simulink model "ReceiveAndUnpack"  (R2023b)
settings: Solver=FixedStepAuto  StartTime=0.0  StopTime=inf  FixedStep=0.01  RelTol=1e-3  EnableMultiTasking=on
libraries: GenericTarget x1, UDPTouchpad x1
settings Model: Creator=damerius  LastModifiedBy=Scythe
settings SolverCC: ConcurrentTasks=on  AlgebraicLoopSolver=TrustRegion  PositivePriorityOrder=on
settings DataIOCC: SaveOutput=off  SignalLogging=off  DSMLogging=off  SaveTime=off  ReturnWorkspaceOutputs=off
settings OptimizationCC: DefaultParameterBehavior=Inlined  ReuseModelBlockBuffer=off  ZeroExternalMemoryAtStartup=off  ZeroInternalMemoryAtStartup=off  SimCompilerOptimization=on
settings DebuggingCC: UnconnectedInputMsg=warning  UnconnectedOutputMsg=warning  UnconnectedLineMsg=warning
settings HardwareCC: ProdBitPerLong=64  ProdHWDeviceType=Intel->x86-64 (Linux 64)
settings ModelReferenceCC: EnableRefExpFcnMdlSchedulingChecks=on
settings SFSimCC: SimParseCustomCode=off  SimGenImportedTypeDefs=on  SimTargetLang=C++
settings RTWCC: GenCodeOnly=on  PackageGeneratedCodeAndArtifacts=on  PackageName=PackNGo  RTWVerbose=off  BuildConfiguration=Faster Runs  TargetLang=C++  DLArmComputeVersion=19.05
settings CodeAppCC: ForceParamTrailComments=on  MaxIdLength=95  MATLABSourceComments=on  UseSimReservedNames=on
settings GRTTargetCC: TargetLangStandard=C++11 (ISO)  GenerateFullHeader=off  MatFileLogging=off  CodeInterfacePackaging=C++ class

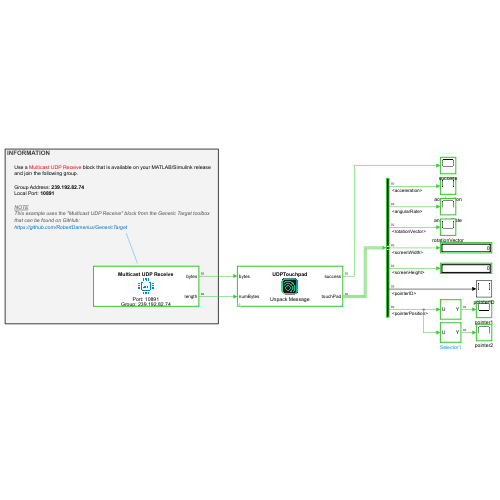
[thumbnail: Simulink's stored preview of the top-level diagram]
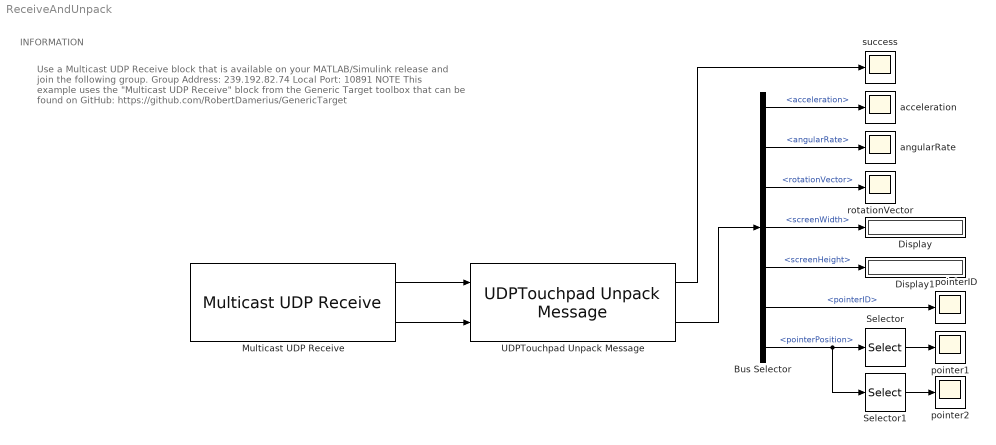
== system ReceiveAndUnpack ==
  note: INFORMATION
  note: Use a Multicast UDP Receive block that is available on your MATLAB/Simulink release
      | and join the following group.
      |
      | Group Address: 239.192.82.74
      | Local Port: 10891
      |
      | NOTE
      | This example uses the "Multicast UDP Receive" block from the Generic Target toolbox
      | that can be found on GitHub:
      | https://github.com/RobertDamerius/GenericTarget
  Bus Selector : BusSelector  OutputSignals=acceleration,angularRate,rotationVector,screenWidth,screenHeight,pointerID,pointerPosition
  Display : Display
  Display1 : Display
  Multicast UDP Receive : GenericTarget/Interface/Multicast UDP Receive  showDetails=off  interfacePortRX=10891  groupIP=[239,192,82,74]  interfaceJoinIP=[0,0,0,0]  interfaceJoinName=''  priorityThread=90  ipFilter=[0,0,0,0]  countAsDiscarded=on  timestampSource=Model Execution Time (default)  rxBufferSize=256  maxNumMessages=1  bufferStrategy=Discard oldest message  SampleTime=0.01
      settings: SourceProductName=Generic Target
  Selector : Selector  NumberOfDimensions=2  InputPortWidth=3  IndexOptions=Select all,Index vector (dialog)  Indices=[1 3],1  OutputSizes=1,1
  Selector1 : Selector  NumberOfDimensions=2  InputPortWidth=3  IndexOptions=Select all,Index vector (dialog)  Indices=[1 3],2  OutputSizes=1,1
  UDPTouchpad Unpack Message : UDPTouchpad/UDPTouchpad Unpack Message
  acceleration : Scope
  angularRate : Scope
  pointer1 : Scope
  pointer2 : Scope
  pointerID : Scope
  rotationVector : Scope
  success : Scope
  wires:
  Multicast UDP Receive/1 -> UDPTouchpad Unpack Message/1
  Multicast UDP Receive/2 -> UDPTouchpad Unpack Message/2
  UDPTouchpad Unpack Message/2 -> Bus Selector/1
  Bus Selector/1 -> acceleration/1  "<acceleration>"
  Bus Selector/2 -> angularRate/1  "<angularRate>"
  Bus Selector/4 -> Display/1  "<screenWidth>"
  Bus Selector/5 -> Display1/1  "<screenHeight>"
  Bus Selector/7 -> Selector1/1, Selector/1  "<pointerPosition>"
  Selector/1 -> pointer1/1
  UDPTouchpad Unpack Message/1 -> success/1
  Selector1/1 -> pointer2/1
  Bus Selector/3 -> rotationVector/1  "<rotationVector>"
  Bus Selector/6 -> pointerID/1  "<pointerID>"
